simulink model "Un_grad_de_libertad"  (R2021a)
settings: Solver=VariableStepAuto  StartTime=0.0  StopTime=15  RelTol=1e-3
settings Model: Creator=Santiago  LastModifiedBy=Santiago

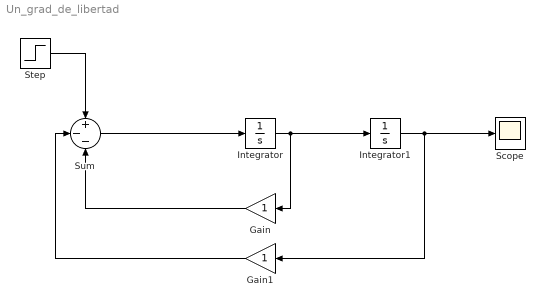
== system Un_grad_de_libertad ==
  Gain : Gain  Gain=1
  Gain1 : Gain  Gain=1
  Integrator : Integrator
  Integrator1 : Integrator
  Scope : Scope
  Step : Step  SampleTime=0
  Sum : Sum  Inputs=+--
  wires:
  Gain1/1 -> Sum/2
  Gain/1 -> Sum/3
  Integrator/1 -> Integrator1/1, Gain/1
  Integrator1/1 -> Scope/1, Gain1/1
  Sum/1 -> Integrator/1
  Step/1 -> Sum/1
